simulink model "rlOvertakeTwoCars"  (R2022b)
settings: Solver=ode45  StartTime=0.0  StopTime=inf  FixedStep=0.001  RelTol=5e-3
PreLoadFcn:
  | setUpModel
PostLoadFcn:
  | setUpMain
model workspace (MAT data in the model file):
  firstWarning = 0
  originalScenarioChecksum = 'F73A6DA3C723D3CA73A6F931B7A52A9C'
values from neighbouring files (symbols this model uses):
  accel_vec = (-4:0.5:4)'    [setUpModel.m]
  amax = 3    [setUpMain.m]
  amin = -3    [setUpMain.m]
  dyNorm = [dyNorm 1.1]    [setUpSlipstream.m]
  e1_initial = 0    [setUpMain.m]
  e2_initial = 0    [setUpMain.m]
  L = data.ActorSpecifications.Length    [setUpModel.m]
  psi_o1 = 0.0058 * (pi/180)    (= 0.000101229096616)    [setUpModel.m]
  psi_o2 = 0.3528 *(pi/180)    (= 0.00615752160104)    [setUpModel.m]
  ry = [ry 0]    [setUpSlipstream.m]
  ssSwitch = 1    [setUpSlipstream.m]
  tolpsi = 10 * pi/180    (= 0.174532925199)    [setUpSlipstream.m]
  toly = 1.2*W /2    [setUpSlipstream.m]
  Ts = 0.1    [setUpMPC.m]
  TsRL = Ts    [setUpRLEnv.m]
  umax = 0.3    [setUpMain.m]
  umin = -0.3    [setUpMain.m]
  v_o1 = highSpeed1    (= 35)    [setUpModel.m]
  v_o2 = highSpeed2    (= 36)    [setUpModel.m]
  vel1 = highSpeed1 * ones(length(xlt),length(ylt))    [setUpModel.m]
  vel2 = highSpeed2 * ones(length(xlt),length(ylt))    [setUpModel.m]
  vel_vec = 0:2:20    [setUpModel.m]
  W = data.ActorSpecifications(1,1).Width    [setUpSlipstream.m]
  X_o1 = xRef1(1)    [setUpModel.m]
  X_o2 = xRef2(1)    [setUpModel.m]
  xFollow = [0 x1 xFollow 60]    [setUpSlipstream.m]
  xLead = [0 -x0 xLead]    [setUpSlipstream.m]
  xlt = -250:10:200    [setUpModel.m]
  Y_o1 = yRef1(1)    [setUpModel.m]
  Y_o2 = yRef2(1)    [setUpModel.m]
  yFollow = [c y1 yFollow 1]    [setUpSlipstream.m]
  yLead = [c y0 yLead]    [setUpSlipstream.m]
  ylt = -150:10:100    [setUpModel.m]
undefined symbols (not defined in the file or in its folder): curvature1, curvature2, deg, DiscIntNeverNeededParam, gradbp1, gradbp2, psi, rad, s, v_o, x_colpen, x_o, y_colpen, Z_colpen
libraries: simulink x26, autolibsharedcommon x22, autolibutils x10, autolibshared x10, vehdynlibtirecommon x8, drivingscenarioandsensors x4, autolibpowerinfoutils x4, sharedtransform x4, aerolibconvert2 x2, simulink_extras x2, vehdynlibtire x2, mpcadaslib x1
(part 2 of 8)

== system rlOvertakeTwoCars/Obs // Reward 9-6 ==
  xgap : Inport
  ygap : Inport  Port=2
  v_lead : Inport  Port=3
  v_ego : Inport  Port=4
  v_ref : Inport  Port=5
  e1 : Inport  Port=6
  e2 : Inport  Port=7
  e1dot : Inport  Port=8
  e2dot : Inport  Port=9
  accel : Inport  Port=10
  steer : Inport  Port=11
  collided : Inport  Port=12
  A : Gain  Gain=0
  Abs : Abs  SaturateOnIntegerOverflow=off
  B : Gain  Gain=2000
  Compare To Constant : simulink/Logic and Bit Operations/Compare To Constant  relop=<=  const=6  OutDataTypeStr=boolean
  E : Gain  Gain=2000
  Gain : Gain  Gain=1/TsRL
  Gain1 : Gain  Gain=20
  Gain2 : Gain  Gain=1/TsRL
  Gain3 : Gain  Gain=1/TsRL
  Goto1 : Goto  Commented=on  GotoTag=p_col  TagVisibility=global
  H : Gain
  Integrator : Integrator
  Integrator1 : Integrator
  Integrator2 : Integrator
  Logical Operator1 : Logic  Operator=OR  Inputs=3  AllPortsSameDT=off  OutDataTypeStr=boolean
  Overtaking : Subsystem
  Path following : Subsystem
  Scope : Scope  NumInputPorts=3
  Scope1 : Scope  NumInputPorts=3
  Scope2 : Scope  NumInputPorts=2
  Subsystem : Subsystem
  Subsystem2 : Subsystem
  Sum : Sum  Inputs=--++
  Sum1 : Sum  Inputs=+++
  Sum2 : Sum
  Zone collision penalty : Lookup_n-D  Commented=on  BreakpointsForDimension1=y_colpen  BreakpointsForDimension2=x_colpen  Table=Z_colpen  ExtrapMethod=Clip  InternalRulePriority=Speed  RndMeth=Simplest
      settings: InputPortMap=u0,u1
      mask Display:
      | image("LookupTable.PNG")
      | port_label('input', 1, 'y')
      | port_label('input', 2, 'x')
      | port_label('output', 1, 'p_col')
  obs : Outport  VectorParamsAs1DForOutWhenUnconnected=off
  Reward : Outport  Port=2  VectorParamsAs1DForOutWhenUnconnected=off
  isDone : Outport  Port=3  VectorParamsAs1DForOutWhenUnconnected=off
  tag scope: onTrack=global
  wires:
  Zone collision penalty/1 -> Sum1/3, Goto1/1
  E/1 -> Sum/2
  Subsystem2/2(failCollided) -> Logical Operator1/2, E/1
  Overtaking/1(r_ot) -> Integrator2/1, Scope1/3, Sum1/2
  B/1 -> Sum/4
  Subsystem2/4(overtakeSuccess) -> B/1
  [ry2] -> Overtaking/1(ry)
  Path following/1(r_pf) -> H/1
  e2dot/1 -> Subsystem/6(e2dot)
  e1/1 -> Abs/1, Path following/2(e1), Subsystem/3(e1), Subsystem2/2(e1)
  e2/1 -> Subsystem/4(e2), Path following/3(e2), Subsystem2/3(e2)
  v_lead/1 -> Subsystem/7(v_lead)
  xgap/1 -> Subsystem/8(xgap), Subsystem2/4(xgap), Zone collision penalty/2, Overtaking/2(xgap)
  Subsystem/1(obs) -> obs/1
  e1dot/1 -> Subsystem/5(e1dot)
  Gain1/1 -> Sum/1
  Abs/1 -> Compare To Constant/1
  Compare To Constant/1 -> [onTrack]
  collided/1 -> Subsystem2/5(collided)
  v_ref/1 -> Subsystem/2(v_ref)
  ygap/1 -> Overtaking/3(ygap), Subsystem/9(ygap), Zone collision penalty/1
  Subsystem/2(v_err) -> Path following/1(v_err), Scope2/2
  steer/1 -> Path following/4(steer)
  accel/1 -> Path following/5(accel)
  Logical Operator1/1 -> isDone/1
  v_ego/1 -> Subsystem2/1(v_ego), Scope2/1, Subsystem/1(v_ego)
  Subsystem2/1(fail) -> Logical Operator1/1, Gain1/1
  Subsystem2/3(completeCourse) -> A/1, Logical Operator1/3
  A/1 -> Sum/3
  Sum2/1 -> Reward/1
  Sum/1 -> Sum2/1
  Sum1/1 -> Scope1/1, Integrator/1, Sum2/2
  Gain/1 -> Scope/1
  Integrator/1 -> Gain/1
  Integrator1/1 -> Gain2/1
  Integrator2/1 -> Gain3/1
  Gain2/1 -> Scope/2
  Gain3/1 -> Scope/3
  H/1 -> Integrator1/1, Scope1/2, Sum1/1

== system rlOvertakeTwoCars/Pedal mapping ==
  xdot : Inport
  AccelerationCmd : Inport  Port=2
  2-D Lookup Table : Lookup_n-D  BreakpointsForDimension1=vel_vec  BreakpointsForDimension2=accel_vec  Table=pedal_map'  InternalRulePriority=Speed  RndMeth=Simplest
      settings: InputPortMap=u0,u1
  Dead Zone1 : DeadZone  LowerValue=-0.001  UpperValue=0.001
  Dead Zone2 : DeadZone  LowerValue=-0.001  UpperValue=0.001
  Gain : Gain  Gain=-1
  Saturation : Saturate  UpperLimit=1  LowerLimit=0
  Saturation1 : Saturate  UpperLimit=0  LowerLimit=-1
  Accel : Outport
  Decel : Outport  Port=2
  wires:
  Dead Zone1/1 -> Accel/1  "Accel"
  Dead Zone2/1 -> Decel/1  "Decel"
  xdot/1 -> 2-D Lookup Table/1
  Saturation/1 -> Dead Zone1/1
  AccelerationCmd/1 -> 2-D Lookup Table/2
  2-D Lookup Table/1 -> Saturation/1, Saturation1/1
  Gain/1 -> Dead Zone2/1
  Saturation1/1 -> Gain/1

== system rlOvertakeTwoCars/Powertrain & Driveline ==
  note: needs x4
  note: Vehicle Feedback
  note: Powertrain & Driveline
  note: Brakes
  note: Longitudinal Command Logic
  Acc : Inport
  Decel : Inport  Port=2
  Friction : Inport  Port=3
  VehFdbk : Inport  Port=4
  Brake System : Subsystem
  Brakes and Wheels : Subsystem  TreatAsAtomicUnit=on
      mask Display: image('vdbslibwhls.png');
  Bus Selector1 : BusSelector  OutputSignals=BdyFrm.Forces.Tires.FrntTires.Lft.Fz,BdyFrm.Forces.Tires.FrntTires.Rght.Fz,BdyFrm.Forces.Tires.RearTires.Lft.Fz,BdyFrm.Forces.Tires.RearTires.Rght.Fz
  Bus Selector2 : BusSelector  OutputSignals=BdyFrm.Cg.Vel.xdot  OutputAsBus=on
  Bus Selector3 : BusSelector  OutputSignals=BdyFrm.FrntAxl.Steer.WhlAngFL,BdyFrm.FrntAxl.Steer.WhlAngFR,BdyFrm.RearAxl.Steer.WhlAngRL,BdyFrm.RearAxl.Steer.WhlAngRR  OutputAsBus=on
  Bus Selector4 : BusSelector  OutputSignals=BdyFrm.Cg.AngVel.r
  Bus to Vector : BusToVector
  Constant : Constant  Value=-1
  Constant1 : Constant  Value=-1
  Motor and Differential : Subsystem
  Mux1 : Mux
  Selector : Selector  InputPortWidth=1  IndexOptions=Index vector (dialog)  Indices=[1 1 1 1]  OutputSizes=1
  Signal Specification : SignalSpecification  Unit=km/hr
  Suspension : autolibutils/Cont LPF  wc=10*pi*2  AbsoluteTolerance=auto  aMode=2
  Switch1 : Switch  Criteria=u2 > Threshold  SaturateOnIntegerOverflow=off  InputSameDT=off
  Switch2 : Switch  Criteria=u2 > Threshold  SaturateOnIntegerOverflow=off  InputSameDT=off
  Terminator : Terminator
  Terminator1 : Terminator
  Unit Conversion : UnitConversion
  Vehicle to Tire : Subsystem
  Front Force : Outport  VectorParamsAs1DForOutWhenUnconnected=off
  Rear Force : Outport  Port=2  VectorParamsAs1DForOutWhenUnconnected=off
  wires:
  Vehicle to Tire/2(WhlVel) -> Brakes and Wheels/4(Vy)
  Vehicle to Tire/1(WhlVelx) -> Brakes and Wheels/3(Vx)
  Brakes and Wheels/1(AxlPwr) -> Terminator1/1
  Brakes and Wheels/4(RearF) -> Rear Force/1
  Brakes and Wheels/3(FrontF) -> Front Force/1
  Brakes and Wheels/2(Omega) -> [Omega]
  VehFdbk/1 -> Vehicle to Tire/1(VehFdbk), Bus Selector3/1, Bus Selector1/1, Bus Selector4/1, Bus Selector2/1
  Selector/1 -> Brakes and Wheels/7(YawRate)
  Bus Selector4/1 -> Selector/1  "<r>"
  Friction/1 -> Brakes and Wheels/8(Friction)
  Signal Specification/1 -> Terminator/1
  Unit Conversion/1 -> Signal Specification/1
  Bus Selector2/1 -> Unit Conversion/1
  Brake System/1(Prs) -> Brakes and Wheels/2(BrkPrs)
  Switch2/1 -> Brake System/1(Decc)  "Decc"
  Bus Selector1/4 -> Mux1/4  "<Fz>"
  Bus Selector1/3 -> Mux1/3  "<Fz>"
  Bus Selector1/2 -> Mux1/2  "<Fz>"
  Bus Selector1/1 -> Mux1/1  "<Fz>"
  Suspension/1 -> Brakes and Wheels/6(Fz)
  Mux1/1 -> Suspension/1
  Bus to Vector/1 -> Brakes and Wheels/5(WhlAng), Vehicle to Tire/2(WhlAng)
  Bus Selector3/1 -> Bus to Vector/1
  Acc/1 -> Switch1/3
  Decel/1 -> Switch2/1, Switch2/2, Switch1/2
  Switch1/1 -> Motor and Differential/1(APP)  "Acc"
  Motor and Differential/1(Axle Torque) -> Brakes and Wheels/1(AxlTrq)
  Constant1/1 -> Switch1/1
  [Omega] -> Motor and Differential/2(Omega)  "Omega"
  Constant/1 -> Switch2/3

== system rlOvertakeTwoCars/Powertrain & Driveline Ego ==
  note: needs x4
  note: Vehicle Feedback
  note: Powertrain & Driveline
  note: Brakes
  note: Longitudinal Command Logic
  Acc : Inport
  Decel : Inport  Port=2
  Friction : Inport  Port=3
  VehFdbk : Inport  Port=4
  Brake System : Subsystem
  Brakes and Wheels : Subsystem  TreatAsAtomicUnit=on
      mask Display: image('vdbslibwhls.png');
  Bus Selector1 : BusSelector  OutputSignals=BdyFrm.Forces.Tires.FrntTires.Lft.Fz,BdyFrm.Forces.Tires.FrntTires.Rght.Fz,BdyFrm.Forces.Tires.RearTires.Lft.Fz,BdyFrm.Forces.Tires.RearTires.Rght.Fz
  Bus Selector2 : BusSelector  OutputSignals=BdyFrm.Cg.Vel.xdot  OutputAsBus=on
  Bus Selector3 : BusSelector  OutputSignals=BdyFrm.FrntAxl.Steer.WhlAngFL,BdyFrm.FrntAxl.Steer.WhlAngFR,BdyFrm.RearAxl.Steer.WhlAngRL,BdyFrm.RearAxl.Steer.WhlAngRR  OutputAsBus=on
  Bus Selector4 : BusSelector  OutputSignals=BdyFrm.Cg.AngVel.r
  Bus to Vector : BusToVector
  Constant : Constant  Value=-1
  Constant1 : Constant  Value=-1
  Motor and Differential : Subsystem
  Mux1 : Mux
  Selector : Selector  InputPortWidth=1  IndexOptions=Index vector (dialog)  Indices=[1 1 1 1]  OutputSizes=1
  Signal Specification : SignalSpecification  Unit=km/hr
  Suspension : autolibutils/Cont LPF  wc=10*pi*2  AbsoluteTolerance=auto  aMode=2
  Switch1 : Switch  Criteria=u2 > Threshold  SaturateOnIntegerOverflow=off  InputSameDT=off
  Switch2 : Switch  Criteria=u2 > Threshold  SaturateOnIntegerOverflow=off  InputSameDT=off
  Terminator : Terminator
  Terminator1 : Terminator
  Unit Conversion : UnitConversion
  Vehicle to Tire : Subsystem
  Front Force : Outport  VectorParamsAs1DForOutWhenUnconnected=off
  Rear Force : Outport  Port=2  VectorParamsAs1DForOutWhenUnconnected=off
  wires:
  Vehicle to Tire/2(WhlVel) -> Brakes and Wheels/4(Vy)
  Vehicle to Tire/1(WhlVelx) -> Brakes and Wheels/3(Vx)
  Brakes and Wheels/1(AxlPwr) -> Terminator1/1
  Brakes and Wheels/4(RearF) -> Rear Force/1
  Brakes and Wheels/3(FrontF) -> Front Force/1
  Brakes and Wheels/2(Omega) -> [Omega]
  VehFdbk/1 -> Vehicle to Tire/1(VehFdbk), Bus Selector3/1, Bus Selector1/1, Bus Selector4/1, Bus Selector2/1
  Selector/1 -> Brakes and Wheels/7(YawRate)
  Bus Selector4/1 -> Selector/1  "<r>"
  Friction/1 -> Brakes and Wheels/8(Friction)
  Signal Specification/1 -> Terminator/1
  Unit Conversion/1 -> Signal Specification/1
  Bus Selector2/1 -> Unit Conversion/1
  Brake System/1(Prs) -> Brakes and Wheels/2(BrkPrs)
  Switch2/1 -> Brake System/1(Decc)  "Decc"
  Bus Selector1/4 -> Mux1/4  "<Fz>"
  Bus Selector1/3 -> Mux1/3  "<Fz>"
  Bus Selector1/2 -> Mux1/2  "<Fz>"
  Bus Selector1/1 -> Mux1/1  "<Fz>"
  Suspension/1 -> Brakes and Wheels/6(Fz)
  Mux1/1 -> Suspension/1
  Bus to Vector/1 -> Brakes and Wheels/5(WhlAng), Vehicle to Tire/2(WhlAng)
  Bus Selector3/1 -> Bus to Vector/1
  Acc/1 -> Switch1/3
  Decel/1 -> Switch2/1, Switch2/2, Switch1/2
  Switch1/1 -> Motor and Differential/1(APP)  "Acc"
  Motor and Differential/1(Axle Torque) -> Brakes and Wheels/1(AxlTrq)
  Constant1/1 -> Switch1/1
  [Omega] -> Motor and Differential/2(Omega)  "Omega"
  Constant/1 -> Switch2/3

== system rlOvertakeTwoCars/Relative distance (Ego from Lead) ==
  pos1 : Inport
  psi1 : Inport  Port=2
  pos2 : Inport  Port=3
  Add : Sum  Inputs=-+
  Add1 : Sum  Inputs=-+
  Add2 : Sum
  Add3 : Sum  Inputs=+-
  Demux : Demux  Outputs=2
  Demux1 : Demux  Outputs=2
  Product{,1..3} (4 alike) : Product
  SinCos : Trigonometry  Operator=sincos
  dx : Outport
  dy : Outport  Port=2
  wires:
  Add2/1 -> dx/1
  Product/1 -> Add2/1
  psi1/1 -> SinCos/1
  Demux1/2 -> Add/2  "y2"
  Product3/1 -> Add3/2
  SinCos/1 -> Product1/1, Product3/1
  Add/1 -> Product1/2, Product2/2  "y2-y1"
  Product2/1 -> Add3/1
  SinCos/2 -> Product/1, Product2/1
  Add3/1 -> dy/1
  Demux/1 -> Add1/1  "x1"
  Product1/1 -> Add2/2
  Demux/2 -> Add/1  "y1"
  Demux1/1 -> Add1/2  "x2"
  Add1/1 -> Product3/2, Product/2  "x2-x1"
  pos1/1 -> Demux/1
  pos2/1 -> Demux1/1

== system rlOvertakeTwoCars/Sensor & road ==
  xdot : Inport
  Curvature lookup : Lookup_n-D  NumberOfTableDimensions=1  BreakpointsForDimension1=gradbp2  Table=curvature2  InterpMethod=Cubic spline  ExtrapMethod=Clip  InternalRulePriority=Speed  RndMeth=Simplest
  Error calculation : Subsystem
  Initial lateral deviation : Constant  Value=e1_initial
  Initial relative yaw angle : Constant  Value=e2_initial
  Integrator : Integrator
  Lateral deviation : Outport
  Relative yaw angle : Outport  Port=2
  e1_dot : Outport  Port=3
  e2_dot : Outport  Port=4
  wires:
  Error calculation/1(Lateral deviation) -> Lateral deviation/1
  Curvature lookup/1 -> Error calculation/4(Curvature)  "rho"
  Error calculation/2(Relative yaw angle) -> Relative yaw angle/1
  Initial lateral deviation/1 -> Error calculation/6(Initial lateral deviation)
  xdot/1 -> Error calculation/1(Longitudinal velocity), Integrator/1
  Initial relative yaw angle/1 -> Error calculation/5(Initial relative yaw angle)
  [ydot2] -> Error calculation/2(Lateral velocity)
  Error calculation/3(e1_dot) -> e1_dot/1
  Integrator/1 -> Curvature lookup/1  "distance"
  Error calculation/4(e2_dot) -> e2_dot/1
  [yawrate2] -> Error calculation/3(Yaw rate)

== system rlOvertakeTwoCars/Slipstream enable ==
  psi1 : Inport
  psi2 : Inport  Port=2
  dy : Inport  Port=3
  AND : Logic  Inputs=3  IconShape=distinctive  AllPortsSameDT=off  OutDataTypeStr=boolean
  Abs : Abs  SaturateOnIntegerOverflow=off
  Abs1 : Abs  SaturateOnIntegerOverflow=off
  Add : Sum  Inputs=+-
  Compare To Constant : simulink/Logic and Bit Operations/Compare To Constant  relop=<=  const=tolpsi  OutDataTypeStr=boolean
  Compare To Constant1 : simulink/Logic and Bit Operations/Compare To Constant  relop=<=  const=toly  OutDataTypeStr=boolean
  Constant : Constant  Value=ssSwitch
  Gain : Gain  Gain=1/(W/2)
  tag scope: SsOn=global, dyNorm=global
  wires:
  Abs/1 -> Compare To Constant/1
  dy/1 -> Abs1/1
  Compare To Constant1/1 -> AND/3
  psi2/1 -> Add/1
  Compare To Constant/1 -> AND/2
  psi1/1 -> Add/2
  Gain/1 -> [dyNorm]
  Abs1/1 -> Gain/1, Compare To Constant1/1
  Add/1 -> Abs/1
  Constant/1 -> AND/1
  AND/1 -> [SsOn]

== system rlOvertakeTwoCars/Steering EMA filter ==
  steer : Inport
  Demux3 : Demux  Outputs=2
  Discrete Filter : DiscreteFilter  Numerator=[0.05]  Denominator=[1 0.95]
  Switch : Switch  Criteria=u2 > Threshold  SaturateOnIntegerOverflow=off  InputSameDT=off
  Terminator5 : Terminator
  delta : Outport
  wires:
  steer/1 -> Switch/3, Discrete Filter/1
  [pos2] -> Demux3/1
  Switch/1 -> delta/1
  Discrete Filter/1 -> Switch/1
  Demux3/2 -> Switch/2  "y2"
  Demux3/1 -> Terminator5/1

== system rlOvertakeTwoCars/Stop Logic ==
  distance : Inport
  Constant : Constant
  Constant3 : Constant  Value=0
  Integrator : Integrator
  Switch : Switch  Threshold=gradbp2(end)+20  SaturateOnIntegerOverflow=off  InputSameDT=off
  stop : Outport
  wires:
  Switch/1 -> stop/1
  Constant3/1 -> Switch/3
  distance/1 -> Integrator/1
  Constant/1 -> Switch/1
  Integrator/1 -> Switch/2

== system rlOvertakeTwoCars/Subsystem ==
  In1 : Inport
  Bus Selector : BusSelector  OutputSignals=InertFrm.Cg.Disp.X,InertFrm.Cg.Disp.Y,InertFrm.Cg.Ang.psi,BdyFrm.Cg.Acc.xddot
  Gain1 : Gain  Gain=180/pi
  Mux : Mux  Inputs=3
  Mux1 : Mux  Inputs=2
  Terminator : Terminator
  Transpose : Math  Operator=transpose  SignedPower=on
  pose : Outport
  pos : Outport  Port=2
  wires:
  Mux/1 -> Transpose/1
  In1/1 -> Bus Selector/1
  Bus Selector/1 -> Mux1/1, Mux/1  "<X>"
  Gain1/1 -> Mux/3
  Bus Selector/2 -> Mux1/2, Mux/2  "<Y>"
  Transpose/1 -> pose/1
  Bus Selector/3 -> Gain1/1  "<psi>"
  Bus Selector/4 -> Terminator/1  "<xddot>"
  Mux1/1 -> pos/1

== system rlOvertakeTwoCars/Subsystem1 ==
  In1 : Inport
  Bus Selector : BusSelector  OutputSignals=InertFrm.Cg.Disp.X,InertFrm.Cg.Disp.Y,InertFrm.Cg.Ang.psi,BdyFrm.Cg.Acc.xddot
  Gain1 : Gain  Gain=180/pi
  Mux : Mux  Inputs=3
  Mux1 : Mux  Inputs=2
  Terminator : Terminator
  Transpose : Math  Operator=transpose  SignedPower=on
  pose : Outport
  pos : Outport  Port=2
  wires:
  Mux/1 -> Transpose/1
  In1/1 -> Bus Selector/1
  Bus Selector/1 -> Mux1/1, Mux/1  "<X>"
  Gain1/1 -> Mux/3
  Bus Selector/2 -> Mux1/2, Mux/2  "<Y>"
  Transpose/1 -> pose/1
  Bus Selector/3 -> Gain1/1  "<psi>"
  Bus Selector/4 -> Terminator/1  "<xddot>"
  Mux1/1 -> pos/1

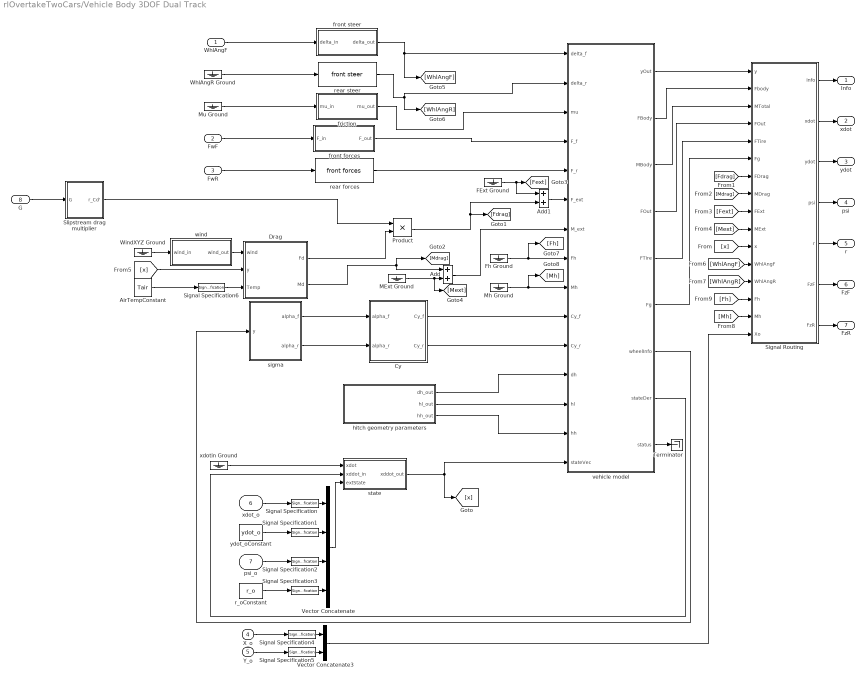
== system rlOvertakeTwoCars/Vehicle Body 3DOF Dual Track ==
  WhlAngF : Inport
  FwF : Inport  Port=2
  FwR : Inport  Port=3
  X_o : Inport  Port=4
  Y_o : Inport  Port=5
  xdot_o : Inport  Port=6
  psi_o : Inport  Port=7
  G : Inport  Port=8
  Add : Sum
  Add1 : Sum
  AirTempConstant : Constant  Value=Tair
  Cy : Subsystem  Variant=on  VariantControlMode=label  LabelModeActiveChoice=2
  Drag : Subsystem
  FExt Ground : Ground
  Fh Ground : Ground
  MExt Ground : Ground
  Mh Ground : Ground
  Mu Ground : Ground
  Product : Product
  Signal Routing : Subsystem  Variant=on  VariantControlMode=label  LabelModeActiveChoice=1
  Signal Specification : SignalSpecification  Unit=m/s
  Signal Specification1 : SignalSpecification  Unit=m/s
  Signal Specification2 : SignalSpecification  Unit=rad
  Signal Specification3 : SignalSpecification  Unit=rad/s
  Signal Specification4 : SignalSpecification  Unit=m
  Signal Specification5 : SignalSpecification  Unit=m
  Signal Specification6 : SignalSpecification  Unit=K
  Slipstream drag multiplier : Subsystem
  Terminator : Terminator
  Vector Concatenate : Concatenate  NumInputs=4
  Vector Concatenate3 : Concatenate
  WhlAngR Ground : Ground
  WindXYZ Ground : Ground
  friction : Subsystem  Variant=on  VariantControlMode=label  LabelModeActiveChoice=2
  front forces : Subsystem  Variant=on  VariantControlMode=label  LabelModeActiveChoice=5
  front steer : Subsystem  Variant=on  VariantControlMode=label  LabelModeActiveChoice=3
  hitch geometry parameters : Subsystem  Variant=on  VariantControlMode=label  LabelModeActiveChoice=3
  r_oConstant : Constant  Value=r_o
  rear forces : autolibshared/Vehicle Body 3DOF Single Track/front forces  SystemSampleTime=-1  LabelModeActiveChoice=5  VariantActivationTime=update diagram  Latency=0  AutoFrameSizeCalculation=off
  rear steer : autolibshared/Vehicle Body 3DOF Single Track/front steer  SystemSampleTime=-1  LabelModeActiveChoice=2  VariantActivationTime=update diagram  Latency=0  AutoFrameSizeCalculation=off
  sigma : Subsystem  Variant=on  VariantControlMode=label  LabelModeActiveChoice=2
  state : Subsystem  Variant=on  VariantControlMode=label  LabelModeActiveChoice=0
  vehicle model : MATLAB Function  TreatAsAtomicUnit=on
  wind : Subsystem  Variant=on  VariantControlMode=label  LabelModeActiveChoice=0
  xdotin Ground : Ground
  ydot_oConstant : Constant  Value=ydot_o
  Info : Outport  VectorParamsAs1DForOutWhenUnconnected=off
  xdot : Outport  Port=2  VectorParamsAs1DForOutWhenUnconnected=off
  ydot : Outport  Port=3  VectorParamsAs1DForOutWhenUnconnected=off
  psi : Outport  Port=4  VectorParamsAs1DForOutWhenUnconnected=off
  r : Outport  Port=5  VectorParamsAs1DForOutWhenUnconnected=off
  FzF : Outport  Port=6  VectorParamsAs1DForOutWhenUnconnected=off
  FzR : Outport  Port=7  VectorParamsAs1DForOutWhenUnconnected=off
  wires:
  AirTempConstant/1 -> Signal Specification6/1
  [Fh] -> Signal Routing/14(Fh)
  [Mh] -> Signal Routing/15(Mh)
  hitch geometry parameters/3(hh_out) -> vehicle model/14(hh)
  hitch geometry parameters/2(hl_out) -> vehicle model/13(hl)
  hitch geometry parameters/1(dh_out) -> vehicle model/12(dh)
  Mh Ground/1 -> [Mh], vehicle model/9(Mh)
  Fh Ground/1 -> [Fh], vehicle model/8(Fh)
  MExt Ground/1 -> Add/2, [Mext]
  FwR/1 -> rear forces/1
  FwF/1 -> front forces/1(F_in)
  xdotin Ground/1 -> state/1(xdot)
  Signal Specification6/1 -> Drag/3(Temp)
  Signal Specification5/1 -> Vector Concatenate3/2
  Signal Specification4/1 -> Vector Concatenate3/1
  Vector Concatenate3/1 -> Signal Routing/16(Xo)
  Signal Specification2/1 -> Vector Concatenate/3
  Signal Specification3/1 -> Vector Concatenate/4
  r_oConstant/1 -> Signal Specification3/1
  Signal Specification1/1 -> Vector Concatenate/2
  ydot_oConstant/1 -> Signal Specification1/1
  Signal Specification/1 -> Vector Concatenate/1
  Vector Concatenate/1 -> state/3(extState)
  [WhlAngR] -> Signal Routing/13(WhlAngR)
  [WhlAngF] -> Signal Routing/12(WhlAngF)
  Signal Routing/4(psi) -> psi/1
  Mu Ground/1 -> friction/1(mu_in)
  WhlAngR Ground/1 -> rear steer/1
  WhlAngF/1 -> front steer/1(delta_in)
  [x] -> Drag/2(y)
  Product/1 -> Add1/2, [Fdrag]
  wind/1(wind_out) -> Drag/1(wind)
  Drag/2(Md) -> [Mdrag], Add/1
  rear forces/1 -> vehicle model/5(F_r)
  front forces/1(F_out) -> vehicle model/4(F_f)
  vehicle model/7(wheelInfo) -> sigma/1(y)
  Signal Routing/1(Info) -> Info/1
  sigma/2(alpha_r) -> Cy/2(alpha_r)
  sigma/1(alpha_f) -> Cy/1(alpha_f)
  rear steer/1 -> vehicle model/2(delta_r), [WhlAngR]
  front steer/1(delta_out) -> [WhlAngF], vehicle model/1(delta_f)
  Cy/2(Cy_r) -> vehicle model/11(Cy_r)
  Cy/1(Cy_f) -> vehicle model/10(Cy_f)
  friction/1(mu_out) -> vehicle model/3(mu)
  vehicle model/8(stateDer) -> state/2(xddot_in)
  vehicle model/1(yOut) -> Signal Routing/1(y)
  Signal Routing/3(ydot) -> ydot/1
  Signal Routing/5(r) -> r/1
  Signal Routing/6(FzF) -> FzF/1
  Signal Routing/7(FzR) -> FzR/1
  Signal Routing/2(xdot) -> xdot/1
  vehicle model/4(FOut) -> Signal Routing/4(FOut)
  state/1(xddot_out) -> vehicle model/15(stateVec), [x]
  [x] -> Signal Routing/11(x)
  vehicle model/9(status) -> Terminator/1
  vehicle model/5(FTire) -> Signal Routing/5(FTire)
  vehicle model/6(Fg) -> Signal Routing/6(Fg)
  [Fext] -> Signal Routing/9(FExt)
  [Fdrag] -> Signal Routing/7(FDrag)
  [Mdrag] -> Signal Routing/8(MDrag)
  [Mext] -> Signal Routing/10(MExt)
  vehicle model/2(FBody) -> Signal Routing/2(Fbody)
  vehicle model/3(MBody) -> Signal Routing/3(MTotal)
  Add/1 -> vehicle model/7(M_ext)
  Add1/1 -> vehicle model/6(F_ext)
  X_o/1 -> Signal Specification4/1
  Y_o/1 -> Signal Specification5/1
  psi_o/1 -> Signal Specification2/1
  xdot_o/1 -> Signal Specification/1
  FExt Ground/1 -> [Fext], Add1/1
  WindXYZ Ground/1 -> wind/1(wind_in)
  Drag/1(Fd) -> Product/2
  G/1 -> Slipstream drag multiplier/1(G)
  Slipstream drag multiplier/1(r_Cd') -> Product/1

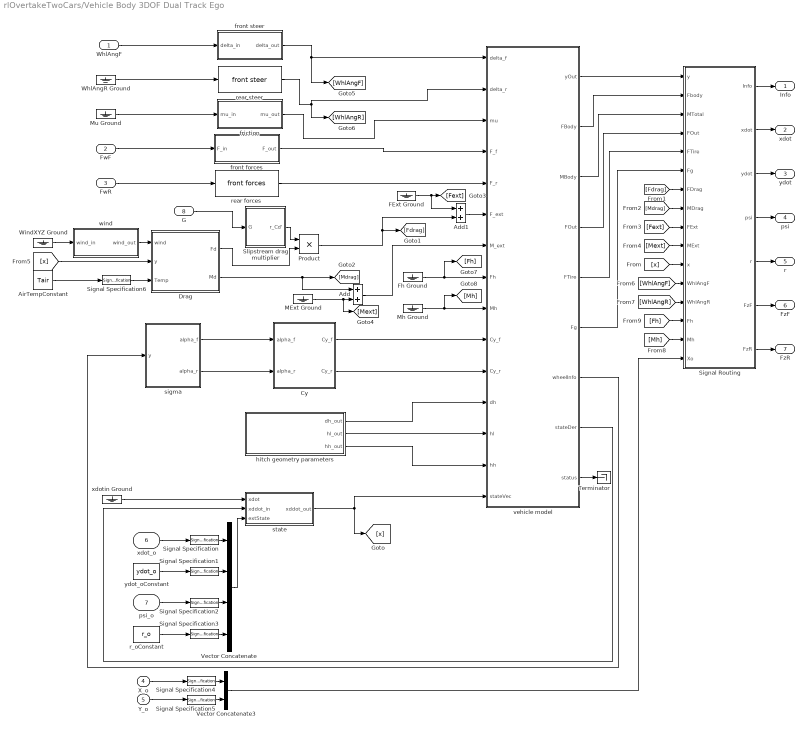
== system rlOvertakeTwoCars/Vehicle Body 3DOF Dual Track Ego ==
  WhlAngF : Inport
  FwF : Inport  Port=2
  FwR : Inport  Port=3
  X_o : Inport  Port=4
  Y_o : Inport  Port=5
  xdot_o : Inport  Port=6
  psi_o : Inport  Port=7
  G : Inport  Port=8
  Add : Sum
  Add1 : Sum
  AirTempConstant : Constant  Value=Tair
  Cy : Subsystem  Variant=on  VariantControlMode=label  LabelModeActiveChoice=2
  Drag : Subsystem
  FExt Ground : Ground
  Fh Ground : Ground
  MExt Ground : Ground
  Mh Ground : Ground
  Mu Ground : Ground
  Product : Product
  Signal Routing : Subsystem  Variant=on  VariantControlMode=label  LabelModeActiveChoice=1
  Signal Specification : SignalSpecification  Unit=m/s
  Signal Specification1 : SignalSpecification  Unit=m/s
  Signal Specification2 : SignalSpecification  Unit=rad
  Signal Specification3 : SignalSpecification  Unit=rad/s
  Signal Specification4 : SignalSpecification  Unit=m
  Signal Specification5 : SignalSpecification  Unit=m
  Signal Specification6 : SignalSpecification  Unit=K
  Slipstream drag multiplier : Subsystem
  Terminator : Terminator
  Vector Concatenate : Concatenate  NumInputs=4
  Vector Concatenate3 : Concatenate
  WhlAngR Ground : Ground
  WindXYZ Ground : Ground
  friction : Subsystem  Variant=on  VariantControlMode=label  LabelModeActiveChoice=2
  front forces : Subsystem  Variant=on  VariantControlMode=label  LabelModeActiveChoice=5
  front steer : Subsystem  Variant=on  VariantControlMode=label  LabelModeActiveChoice=3
  hitch geometry parameters : Subsystem  Variant=on  VariantControlMode=label  LabelModeActiveChoice=3
  r_oConstant : Constant  Value=r_o
  rear forces : autolibshared/Vehicle Body 3DOF Single Track/front forces  SystemSampleTime=-1  LabelModeActiveChoice=5  VariantActivationTime=update diagram  Latency=0  AutoFrameSizeCalculation=off
  rear steer : autolibshared/Vehicle Body 3DOF Single Track/front steer  SystemSampleTime=-1  LabelModeActiveChoice=2  VariantActivationTime=update diagram  Latency=0  AutoFrameSizeCalculation=off
  sigma : Subsystem  Variant=on  VariantControlMode=label  LabelModeActiveChoice=2
  state : Subsystem  Variant=on  VariantControlMode=label  LabelModeActiveChoice=0
  vehicle model : MATLAB Function  TreatAsAtomicUnit=on
  wind : Subsystem  Variant=on  VariantControlMode=label  LabelModeActiveChoice=0
  xdotin Ground : Ground
  ydot_oConstant : Constant  Value=ydot_o
  Info : Outport  VectorParamsAs1DForOutWhenUnconnected=off
  xdot : Outport  Port=2  VectorParamsAs1DForOutWhenUnconnected=off
  ydot : Outport  Port=3  VectorParamsAs1DForOutWhenUnconnected=off
  psi : Outport  Port=4  VectorParamsAs1DForOutWhenUnconnected=off
  r : Outport  Port=5  VectorParamsAs1DForOutWhenUnconnected=off
  FzF : Outport  Port=6  VectorParamsAs1DForOutWhenUnconnected=off
  FzR : Outport  Port=7  VectorParamsAs1DForOutWhenUnconnected=off
  wires:
  AirTempConstant/1 -> Signal Specification6/1
  [Fh] -> Signal Routing/14(Fh)
  [Mh] -> Signal Routing/15(Mh)
  hitch geometry parameters/3(hh_out) -> vehicle model/14(hh)
  hitch geometry parameters/2(hl_out) -> vehicle model/13(hl)
  hitch geometry parameters/1(dh_out) -> vehicle model/12(dh)
  Mh Ground/1 -> [Mh], vehicle model/9(Mh)
  Fh Ground/1 -> [Fh], vehicle model/8(Fh)
  MExt Ground/1 -> Add/2, [Mext]
  FwR/1 -> rear forces/1
  FwF/1 -> front forces/1(F_in)
  xdotin Ground/1 -> state/1(xdot)
  Signal Specification6/1 -> Drag/3(Temp)
  Signal Specification5/1 -> Vector Concatenate3/2
  Signal Specification4/1 -> Vector Concatenate3/1
  Vector Concatenate3/1 -> Signal Routing/16(Xo)
  Signal Specification2/1 -> Vector Concatenate/3
  Signal Specification3/1 -> Vector Concatenate/4
  r_oConstant/1 -> Signal Specification3/1
  Signal Specification1/1 -> Vector Concatenate/2
  ydot_oConstant/1 -> Signal Specification1/1
  Signal Specification/1 -> Vector Concatenate/1
  Vector Concatenate/1 -> state/3(extState)
  [WhlAngR] -> Signal Routing/13(WhlAngR)
  [WhlAngF] -> Signal Routing/12(WhlAngF)
  Signal Routing/4(psi) -> psi/1
  Mu Ground/1 -> friction/1(mu_in)
  WhlAngR Ground/1 -> rear steer/1
  WhlAngF/1 -> front steer/1(delta_in)
  [x] -> Drag/2(y)
  Product/1 -> Add1/2, [Fdrag]
  wind/1(wind_out) -> Drag/1(wind)
  Drag/2(Md) -> Add/1, [Mdrag]
  rear forces/1 -> vehicle model/5(F_r)
  front forces/1(F_out) -> vehicle model/4(F_f)
  vehicle model/7(wheelInfo) -> sigma/1(y)
  Signal Routing/1(Info) -> Info/1
  sigma/2(alpha_r) -> Cy/2(alpha_r)
  sigma/1(alpha_f) -> Cy/1(alpha_f)
  rear steer/1 -> vehicle model/2(delta_r), [WhlAngR]
  front steer/1(delta_out) -> [WhlAngF], vehicle model/1(delta_f)
  Cy/2(Cy_r) -> vehicle model/11(Cy_r)
  Cy/1(Cy_f) -> vehicle model/10(Cy_f)
  friction/1(mu_out) -> vehicle model/3(mu)
  vehicle model/8(stateDer) -> state/2(xddot_in)
  vehicle model/1(yOut) -> Signal Routing/1(y)
  Signal Routing/3(ydot) -> ydot/1
  Signal Routing/5(r) -> r/1
  Signal Routing/6(FzF) -> FzF/1
  Signal Routing/7(FzR) -> FzR/1
  Signal Routing/2(xdot) -> xdot/1
  vehicle model/4(FOut) -> Signal Routing/4(FOut)
  state/1(xddot_out) -> vehicle model/15(stateVec), [x]
  [x] -> Signal Routing/11(x)
  vehicle model/9(status) -> Terminator/1
  vehicle model/5(FTire) -> Signal Routing/5(FTire)
  vehicle model/6(Fg) -> Signal Routing/6(Fg)
  [Fext] -> Signal Routing/9(FExt)
  [Fdrag] -> Signal Routing/7(FDrag)
  [Mdrag] -> Signal Routing/8(MDrag)
  [Mext] -> Signal Routing/10(MExt)
  vehicle model/2(FBody) -> Signal Routing/2(Fbody)
  vehicle model/3(MBody) -> Signal Routing/3(MTotal)
  Add/1 -> vehicle model/7(M_ext)
  Add1/1 -> vehicle model/6(F_ext)
  X_o/1 -> Signal Specification4/1
  Y_o/1 -> Signal Specification5/1
  psi_o/1 -> Signal Specification2/1
  xdot_o/1 -> Signal Specification/1
  FExt Ground/1 -> [Fext], Add1/1
  WindXYZ Ground/1 -> wind/1(wind_in)
  Drag/1(Fd) -> Product/2
  G/1 -> Slipstream drag multiplier/1(G)
  Slipstream drag multiplier/1(r_Cd') -> Product/1

== system rlOvertakeTwoCars/Collision Detector/Corner and car centre 1 ==
  psi1 : Inport
  pos1 : Inport  Port=2
  Add : Sum
  Add1 : Sum
  Add10 : Sum  Inputs=++-
  Add11 : Sum  Inputs=+++
  Add12 : Sum  Inputs=+++
  Add13 : Sum  Inputs=++-
  Add6 : Sum  Inputs=+--
  Add7 : Sum  Inputs=+-+
  Add8 : Sum  Inputs=+-+
  Add9 : Sum  Inputs=+--
  Demux : Demux  Outputs=2
  Gain : Gain  Gain=L/2-1
  Gain2 : Gain  Gain=L/2-1
  Gain3 : Gain  Gain=L/2
  Gain4 : Gain  Gain=L/2
  Gain5 : Gain  Gain=W/2
  Gain6 : Gain  Gain=W/2
  Mux{1..5} (5 alike) : Mux  Inputs=2
  Mux6 : Mux
  SinCos : Trigonometry  Operator=sincos
  c1 : Outport
  corners_v1 : Outport  Port=2
  wires:
  Demux/1 -> Add1/2  "x1"
  Add12/1 -> Mux5/1
  Add13/1 -> Mux5/2
  Add6/1 -> Mux2/1
  Mux2/1 -> Mux6/1
  psi1/1 -> SinCos/1
  Add/1 -> Mux1/2, Add13/1, Add11/1, Add9/1, Add7/1  "yc"
  Mux3/1 -> Mux6/2
  Mux6/1 -> corners_v1/1
  Mux4/1 -> Mux6/3
  Gain3/1 -> Add12/2, Add8/2, Add6/2, Add10/2
  Add11/1 -> Mux4/2
  Add7/1 -> Mux2/2
  Gain6/1 -> Add8/3, Add6/3, Add10/3, Add12/3
  Add9/1 -> Mux3/2
  Add1/1 -> Add12/1, Add10/1, Add8/1, Mux1/1, Add6/1  "xc"
  SinCos/1 -> Gain6/1, Gain4/1, Gain/1  "s"
  Add8/1 -> Mux3/1
  Demux/2 -> Add/2  "y1"
  Gain/1 -> Add1/1
  SinCos/2 -> Gain5/1, Gain3/1, Gain2/1  "c"
  Mux5/1 -> Mux6/4
  Gain2/1 -> Add/1
  Add10/1 -> Mux4/1
  Gain4/1 -> Add13/2, Add11/2, Add9/2, Add7/2
  Gain5/1 -> Add11/3, Add9/3, Add7/3, Add13/3
  Mux1/1 -> c1/1
  pos1/1 -> Demux/1

== system rlOvertakeTwoCars/Collision Detector/Corner and car centre 2 ==
  psi2 : Inport
  pos2 : Inport  Port=2
  Add : Sum
  Add1 : Sum
  Add10 : Sum  Inputs=++-
  Add11 : Sum  Inputs=+++
  Add12 : Sum  Inputs=+++
  Add13 : Sum  Inputs=++-
  Add6 : Sum  Inputs=+--
  Add7 : Sum  Inputs=+-+
  Add8 : Sum  Inputs=+-+
  Add9 : Sum  Inputs=+--
  Demux : Demux  Outputs=2
  Gain : Gain  Gain=L/2-1
  Gain2 : Gain  Gain=L/2-1
  Gain3 : Gain  Gain=L/2
  Gain4 : Gain  Gain=L/2
  Gain5 : Gain  Gain=W/2
  Gain6 : Gain  Gain=W/2
  Mux{1..5} (5 alike) : Mux  Inputs=2
  Mux6 : Mux
  SinCos : Trigonometry  Operator=sincos
  c2 : Outport
  corners_v2 : Outport  Port=2
  wires:
  Demux/1 -> Add1/2
  Add12/1 -> Mux5/1
  Add13/1 -> Mux5/2
  Add6/1 -> Mux2/1
  Mux2/1 -> Mux6/1
  psi2/1 -> SinCos/1
  Add/1 -> Mux1/2, Add13/1, Add11/1, Add9/1, Add7/1  "yc"
  Mux3/1 -> Mux6/2
  Mux6/1 -> corners_v2/1
  Mux4/1 -> Mux6/3
  Gain3/1 -> Add12/2, Add8/2, Add6/2, Add10/2
  Add11/1 -> Mux4/2
  Add7/1 -> Mux2/2
  Gain6/1 -> Add8/3, Add6/3, Add10/3, Add12/3
  Add9/1 -> Mux3/2
  Add1/1 -> Add12/1, Add10/1, Add8/1, Mux1/1, Add6/1  "xc"
  SinCos/1 -> Gain6/1, Gain4/1, Gain/1  "s"
  Add8/1 -> Mux3/1
  Demux/2 -> Add/2
  Gain/1 -> Add1/1
  SinCos/2 -> Gain5/1, Gain3/1, Gain2/1  "c"
  Mux5/1 -> Mux6/4
  Gain2/1 -> Add/1
  Add10/1 -> Mux4/1
  Gain4/1 -> Add13/2, Add11/2, Add9/2, Add7/2
  Gain5/1 -> Add11/3, Add9/3, Add7/3, Add13/3
  Mux1/1 -> c2/1
  pos2/1 -> Demux/1

== system rlOvertakeTwoCars/Collision Detector/Subsystem10 ==
  psi1 : Inport
  c1 : Inport  Port=2
  v2cor3 : Inport  Port=3
  Abs : Abs  SaturateOnIntegerOverflow=off
  Abs1 : Abs  SaturateOnIntegerOverflow=off
  Add : Sum  Inputs=-+
  Add1 : Sum  Inputs=-+
  Add2 : Sum  Inputs=+-
  Add3 : Sum
  Compare To Constant : simulink/Logic and Bit Operations/Compare To Constant  relop=>  const=L/2  OutDataTypeStr=boolean
  Compare To Constant1 : simulink/Logic and Bit Operations/Compare To Constant  relop=>  const=W/2  OutDataTypeStr=boolean
  Demux1 : Demux  Outputs=2
  Demux2 : Demux  Outputs=2
  Gain : Gain  Gain=-1
  NOT : Logic  Operator=NOT  IconShape=distinctive  AllPortsSameDT=off  OutDataTypeStr=boolean
  OR : Logic  Operator=OR  IconShape=distinctive  AllPortsSameDT=off  OutDataTypeStr=boolean
  Product{,1..3} (4 alike) : Product
  SinCos : Trigonometry  Operator=sincos
  collided : Outport
  wires:
  Demux2/1 -> Add1/1
  OR/1 -> NOT/1
  c1/1 -> Demux2/1
  Add1/1 -> Product2/1, Product/1  "dx"
  SinCos/1 -> Product2/2, Product1/2  "s"
  Demux1/1 -> Add1/2  "point0"
  Abs1/1 -> Compare To Constant1/1
  Compare To Constant1/1 -> OR/2
  Demux1/2 -> Add/2  "point1"
  NOT/1 -> collided/1
  Abs/1 -> Compare To Constant/1
  Demux2/2 -> Add/1
  Product/1 -> Add2/1
  v2cor3/1 -> Demux1/1
  psi1/1 -> Gain/1
  Gain/1 -> SinCos/1
  Product2/1 -> Add3/1
  Product3/1 -> Add3/2
  Compare To Constant/1 -> OR/1
  SinCos/2 -> Product3/2, Product/2  "c"
  Add2/1 -> Abs/1  "rot_dx"
  Add3/1 -> Abs1/1  "rot_dy"
  Product1/1 -> Add2/2
  Add/1 -> Product1/1, Product3/1  "dy"

== system rlOvertakeTwoCars/Collision Detector/Subsystem11 ==
  psi1 : Inport
  c1 : Inport  Port=2
  v2cor4 : Inport  Port=3
  Abs : Abs  SaturateOnIntegerOverflow=off
  Abs1 : Abs  SaturateOnIntegerOverflow=off
  Add : Sum  Inputs=-+
  Add1 : Sum  Inputs=-+
  Add2 : Sum  Inputs=+-
  Add3 : Sum
  Compare To Constant : simulink/Logic and Bit Operations/Compare To Constant  relop=>  const=L/2  OutDataTypeStr=boolean
  Compare To Constant1 : simulink/Logic and Bit Operations/Compare To Constant  relop=>  const=W/2  OutDataTypeStr=boolean
  Demux1 : Demux  Outputs=2
  Demux2 : Demux  Outputs=2
  Gain : Gain  Gain=-1
  NOT : Logic  Operator=NOT  IconShape=distinctive  AllPortsSameDT=off  OutDataTypeStr=boolean
  OR : Logic  Operator=OR  IconShape=distinctive  AllPortsSameDT=off  OutDataTypeStr=boolean
  Product{,1..3} (4 alike) : Product
  SinCos : Trigonometry  Operator=sincos
  collided : Outport
  wires:
  Demux2/1 -> Add1/1
  OR/1 -> NOT/1
  c1/1 -> Demux2/1
  Add1/1 -> Product2/1, Product/1  "dx"
  SinCos/1 -> Product2/2, Product1/2  "s"
  Demux1/1 -> Add1/2  "point0"
  Abs1/1 -> Compare To Constant1/1
  Compare To Constant1/1 -> OR/2
  Demux1/2 -> Add/2  "point1"
  NOT/1 -> collided/1
  Abs/1 -> Compare To Constant/1
  Demux2/2 -> Add/1
  Product/1 -> Add2/1
  v2cor4/1 -> Demux1/1
  psi1/1 -> Gain/1
  Gain/1 -> SinCos/1
  Product2/1 -> Add3/1
  Product3/1 -> Add3/2
  Compare To Constant/1 -> OR/1
  SinCos/2 -> Product3/2, Product/2  "c"
  Add2/1 -> Abs/1  "rot_dx"
  Add3/1 -> Abs1/1  "rot_dy"
  Product1/1 -> Add2/2
  Add/1 -> Product1/1, Product3/1  "dy"

== system rlOvertakeTwoCars/Collision Detector/Subsystem3 ==
  psi2 : Inport
  c2 : Inport  Port=2
  v1cor1 : Inport  Port=3
  Abs : Abs  SaturateOnIntegerOverflow=off
  Abs1 : Abs  SaturateOnIntegerOverflow=off
  Add : Sum  Inputs=-+
  Add1 : Sum  Inputs=-+
  Add2 : Sum  Inputs=+-
  Add3 : Sum
  Compare To Constant : simulink/Logic and Bit Operations/Compare To Constant  relop=>  const=L/2  OutDataTypeStr=boolean
  Compare To Constant1 : simulink/Logic and Bit Operations/Compare To Constant  relop=>  const=W/2  OutDataTypeStr=boolean
  Demux1 : Demux  Outputs=2
  Demux2 : Demux  Outputs=2
  Gain : Gain  Gain=-1
  NOT : Logic  Operator=NOT  IconShape=distinctive  AllPortsSameDT=off  OutDataTypeStr=boolean
  OR : Logic  Operator=OR  IconShape=distinctive  AllPortsSameDT=off  OutDataTypeStr=boolean
  Product{,1..3} (4 alike) : Product
  SinCos : Trigonometry  Operator=sincos
  collided : Outport
  wires:
  Demux2/1 -> Add1/1
  OR/1 -> NOT/1
  c2/1 -> Demux2/1
  Add1/1 -> Product2/1, Product/1  "dx"
  SinCos/1 -> Product2/2, Product1/2  "s"
  Demux1/1 -> Add1/2  "point0"
  Abs1/1 -> Compare To Constant1/1
  Compare To Constant1/1 -> OR/2
  Demux1/2 -> Add/2  "point1"
  NOT/1 -> collided/1
  Abs/1 -> Compare To Constant/1
  Demux2/2 -> Add/1
  Product/1 -> Add2/1
  v1cor1/1 -> Demux1/1
  psi2/1 -> Gain/1
  Gain/1 -> SinCos/1
  Product2/1 -> Add3/1
  Product3/1 -> Add3/2
  Compare To Constant/1 -> OR/1
  SinCos/2 -> Product3/2, Product/2  "c"
  Add2/1 -> Abs/1  "rot_dx"
  Add3/1 -> Abs1/1  "rot_dy"
  Product1/1 -> Add2/2
  Add/1 -> Product1/1, Product3/1  "dy"

== system rlOvertakeTwoCars/Collision Detector/Subsystem5 ==
  psi2 : Inport
  c2 : Inport  Port=2
  v1cor2 : Inport  Port=3
  Abs : Abs  SaturateOnIntegerOverflow=off
  Abs1 : Abs  SaturateOnIntegerOverflow=off
  Add : Sum  Inputs=-+
  Add1 : Sum  Inputs=-+
  Add2 : Sum  Inputs=+-
  Add3 : Sum
  Compare To Constant : simulink/Logic and Bit Operations/Compare To Constant  relop=>  const=L/2  OutDataTypeStr=boolean
  Compare To Constant1 : simulink/Logic and Bit Operations/Compare To Constant  relop=>  const=W/2  OutDataTypeStr=boolean
  Demux1 : Demux  Outputs=2
  Demux2 : Demux  Outputs=2
  Gain : Gain  Gain=-1
  NOT : Logic  Operator=NOT  IconShape=distinctive  AllPortsSameDT=off  OutDataTypeStr=boolean
  OR : Logic  Operator=OR  IconShape=distinctive  AllPortsSameDT=off  OutDataTypeStr=boolean
  Product{,1..3} (4 alike) : Product
  SinCos : Trigonometry  Operator=sincos
  collided : Outport
  wires:
  Demux2/1 -> Add1/1
  OR/1 -> NOT/1
  c2/1 -> Demux2/1
  Add1/1 -> Product2/1, Product/1  "dx"
  SinCos/1 -> Product2/2, Product1/2  "s"
  Demux1/1 -> Add1/2  "point0"
  Abs1/1 -> Compare To Constant1/1
  Compare To Constant1/1 -> OR/2
  Demux1/2 -> Add/2  "point1"
  NOT/1 -> collided/1
  Abs/1 -> Compare To Constant/1
  Demux2/2 -> Add/1
  Product/1 -> Add2/1
  v1cor2/1 -> Demux1/1
  psi2/1 -> Gain/1
  Gain/1 -> SinCos/1
  Product2/1 -> Add3/1
  Product3/1 -> Add3/2
  Compare To Constant/1 -> OR/1
  SinCos/2 -> Product3/2, Product/2  "c"
  Add2/1 -> Abs/1  "rot_dx"
  Add3/1 -> Abs1/1  "rot_dy"
  Product1/1 -> Add2/2
  Add/1 -> Product1/1, Product3/1  "dy"

== system rlOvertakeTwoCars/Collision Detector/Subsystem6 ==
  psi2 : Inport
  c2 : Inport  Port=2
  v1cor3 : Inport  Port=3
  Abs : Abs  SaturateOnIntegerOverflow=off
  Abs1 : Abs  SaturateOnIntegerOverflow=off
  Add : Sum  Inputs=-+
  Add1 : Sum  Inputs=-+
  Add2 : Sum  Inputs=+-
  Add3 : Sum
  Compare To Constant : simulink/Logic and Bit Operations/Compare To Constant  relop=>  const=L/2  OutDataTypeStr=boolean
  Compare To Constant1 : simulink/Logic and Bit Operations/Compare To Constant  relop=>  const=W/2  OutDataTypeStr=boolean
  Demux1 : Demux  Outputs=2
  Demux2 : Demux  Outputs=2
  Gain : Gain  Gain=-1
  NOT : Logic  Operator=NOT  IconShape=distinctive  AllPortsSameDT=off  OutDataTypeStr=boolean
  OR : Logic  Operator=OR  IconShape=distinctive  AllPortsSameDT=off  OutDataTypeStr=boolean
  Product{,1..3} (4 alike) : Product
  SinCos : Trigonometry  Operator=sincos
  collided : Outport
  wires:
  Demux2/1 -> Add1/1
  OR/1 -> NOT/1
  c2/1 -> Demux2/1
  Add1/1 -> Product2/1, Product/1  "dx"
  SinCos/1 -> Product2/2, Product1/2  "s"
  Demux1/1 -> Add1/2  "point0"
  Abs1/1 -> Compare To Constant1/1
  Compare To Constant1/1 -> OR/2
  Demux1/2 -> Add/2  "point1"
  NOT/1 -> collided/1
  Abs/1 -> Compare To Constant/1
  Demux2/2 -> Add/1
  Product/1 -> Add2/1
  v1cor3/1 -> Demux1/1
  psi2/1 -> Gain/1
  Gain/1 -> SinCos/1
  Product2/1 -> Add3/1
  Product3/1 -> Add3/2
  Compare To Constant/1 -> OR/1
  SinCos/2 -> Product3/2, Product/2  "c"
  Add2/1 -> Abs/1  "rot_dx"
  Add3/1 -> Abs1/1  "rot_dy"
  Product1/1 -> Add2/2
  Add/1 -> Product1/1, Product3/1  "dy"

== system rlOvertakeTwoCars/Collision Detector/Subsystem7 ==
  psi2 : Inport
  c2 : Inport  Port=2
  v1cor4 : Inport  Port=3
  Abs : Abs  SaturateOnIntegerOverflow=off
  Abs1 : Abs  SaturateOnIntegerOverflow=off
  Add : Sum  Inputs=-+
  Add1 : Sum  Inputs=-+
  Add2 : Sum  Inputs=+-
  Add3 : Sum
  Compare To Constant : simulink/Logic and Bit Operations/Compare To Constant  relop=>  const=L/2  OutDataTypeStr=boolean
  Compare To Constant1 : simulink/Logic and Bit Operations/Compare To Constant  relop=>  const=W/2  OutDataTypeStr=boolean
  Demux1 : Demux  Outputs=2
  Demux2 : Demux  Outputs=2
  Gain : Gain  Gain=-1
  NOT : Logic  Operator=NOT  IconShape=distinctive  AllPortsSameDT=off  OutDataTypeStr=boolean
  OR : Logic  Operator=OR  IconShape=distinctive  AllPortsSameDT=off  OutDataTypeStr=boolean
  Product{,1..3} (4 alike) : Product
  SinCos : Trigonometry  Operator=sincos
  collided : Outport
  wires:
  Demux2/1 -> Add1/1
  OR/1 -> NOT/1
  c2/1 -> Demux2/1
  Add1/1 -> Product2/1, Product/1  "dx"
  SinCos/1 -> Product2/2, Product1/2  "s"
  Demux1/1 -> Add1/2  "point0"
  Abs1/1 -> Compare To Constant1/1
  Compare To Constant1/1 -> OR/2
  Demux1/2 -> Add/2  "point1"
  NOT/1 -> collided/1
  Abs/1 -> Compare To Constant/1
  Demux2/2 -> Add/1
  Product/1 -> Add2/1
  v1cor4/1 -> Demux1/1
  psi2/1 -> Gain/1
  Gain/1 -> SinCos/1
  Product2/1 -> Add3/1
  Product3/1 -> Add3/2
  Compare To Constant/1 -> OR/1
  SinCos/2 -> Product3/2, Product/2  "c"
  Add2/1 -> Abs/1  "rot_dx"
  Add3/1 -> Abs1/1  "rot_dy"
  Product1/1 -> Add2/2
  Add/1 -> Product1/1, Product3/1  "dy"

== system rlOvertakeTwoCars/Collision Detector/Subsystem8 ==
  psi1 : Inport
  c1 : Inport  Port=2
  v2cor1 : Inport  Port=3
  Abs : Abs  SaturateOnIntegerOverflow=off
  Abs1 : Abs  SaturateOnIntegerOverflow=off
  Add : Sum  Inputs=-+
  Add1 : Sum  Inputs=-+
  Add2 : Sum  Inputs=+-
  Add3 : Sum
  Compare To Constant : simulink/Logic and Bit Operations/Compare To Constant  relop=>  const=L/2  OutDataTypeStr=boolean
  Compare To Constant1 : simulink/Logic and Bit Operations/Compare To Constant  relop=>  const=W/2  OutDataTypeStr=boolean
  Demux1 : Demux  Outputs=2
  Demux2 : Demux  Outputs=2
  Gain : Gain  Gain=-1
  NOT : Logic  Operator=NOT  IconShape=distinctive  AllPortsSameDT=off  OutDataTypeStr=boolean
  OR : Logic  Operator=OR  IconShape=distinctive  AllPortsSameDT=off  OutDataTypeStr=boolean
  Product{,1..3} (4 alike) : Product
  SinCos : Trigonometry  Operator=sincos
  collided : Outport
  wires:
  Demux2/1 -> Add1/1
  OR/1 -> NOT/1
  c1/1 -> Demux2/1
  Add1/1 -> Product2/1, Product/1  "dx"
  SinCos/1 -> Product2/2, Product1/2  "s"
  Demux1/1 -> Add1/2  "point0"
  Abs1/1 -> Compare To Constant1/1
  Compare To Constant1/1 -> OR/2
  Demux1/2 -> Add/2  "point1"
  NOT/1 -> collided/1
  Abs/1 -> Compare To Constant/1
  Demux2/2 -> Add/1
  Product/1 -> Add2/1
  v2cor1/1 -> Demux1/1
  psi1/1 -> Gain/1
  Gain/1 -> SinCos/1
  Product2/1 -> Add3/1
  Product3/1 -> Add3/2
  Compare To Constant/1 -> OR/1
  SinCos/2 -> Product3/2, Product/2  "c"
  Add2/1 -> Abs/1  "rot_dx"
  Add3/1 -> Abs1/1  "rot_dy"
  Product1/1 -> Add2/2
  Add/1 -> Product1/1, Product3/1  "dy"

== system rlOvertakeTwoCars/Collision Detector/Subsystem9 ==
  psi1 : Inport
  c1 : Inport  Port=2
  v2cor2 : Inport  Port=3
  Abs : Abs  SaturateOnIntegerOverflow=off
  Abs1 : Abs  SaturateOnIntegerOverflow=off
  Add : Sum  Inputs=-+
  Add1 : Sum  Inputs=-+
  Add2 : Sum  Inputs=+-
  Add3 : Sum
  Compare To Constant : simulink/Logic and Bit Operations/Compare To Constant  relop=>  const=L/2  OutDataTypeStr=boolean
  Compare To Constant1 : simulink/Logic and Bit Operations/Compare To Constant  relop=>  const=W/2  OutDataTypeStr=boolean
  Demux1 : Demux  Outputs=2
  Demux2 : Demux  Outputs=2
  Gain : Gain  Gain=-1
  NOT : Logic  Operator=NOT  IconShape=distinctive  AllPortsSameDT=off  OutDataTypeStr=boolean
  OR : Logic  Operator=OR  IconShape=distinctive  AllPortsSameDT=off  OutDataTypeStr=boolean
  Product{,1..3} (4 alike) : Product
  SinCos : Trigonometry  Operator=sincos
  collided : Outport
  wires:
  Demux2/1 -> Add1/1
  OR/1 -> NOT/1
  c1/1 -> Demux2/1
  Add1/1 -> Product2/1, Product/1  "dx"
  SinCos/1 -> Product2/2, Product1/2  "s"
  Demux1/1 -> Add1/2  "point0"
  Abs1/1 -> Compare To Constant1/1
  Compare To Constant1/1 -> OR/2
  Demux1/2 -> Add/2  "point1"
  NOT/1 -> collided/1
  Abs/1 -> Compare To Constant/1
  Demux2/2 -> Add/1
  Product/1 -> Add2/1
  v2cor2/1 -> Demux1/1
  psi1/1 -> Gain/1
  Gain/1 -> SinCos/1
  Product2/1 -> Add3/1
  Product3/1 -> Add3/2
  Compare To Constant/1 -> OR/1
  SinCos/2 -> Product3/2, Product/2  "c"
  Add2/1 -> Abs/1  "rot_dx"
  Add3/1 -> Abs1/1  "rot_dy"
  Product1/1 -> Add2/2
  Add/1 -> Product1/1, Product3/1  "dy"

== system rlOvertakeTwoCars/MPC Based Controller/Pedal map ==
  note: This 2-D Lookup Table was created using a for-loop and then normalizing. This is required because the output of the MPC controller is acceleration (m/s^2), but the powertrain model uses pedal commands from 0-1.
      |
      | Here are the steps in the script to create the table:
      |
      | 1.) The for-loop is used to calculate the required torque (Nm) from the powertrain.
      | 2.) The positive torque values are normalized based on peak positive motor torque, and the negative torques are normalized based on the peak brake pressure. This results in a pedal map with values of -1 to 1.
      |
      | This map required two values to be calibrated.
      |
      | This is a simple linearized map, but this can be altered for better drivability.
  note: The saturation blocks ensure the acceleration limits are kept at ±1.
  note: The 'Dead Zone' blocks is used to ensure that the pedal command is zero.
  vx : Inport
  a : Inport  Port=2
  Dead Zone1 : DeadZone  LowerValue=-0.001  UpperValue=0.001
  Dead Zone2 : DeadZone  LowerValue=-0.001  UpperValue=0.001
  Gain : Gain  Gain=-1
  Pedal map : Lookup_n-D  BreakpointsForDimension1=vel_vec  BreakpointsForDimension2=accel_vec  Table=pedal_map'  InternalRulePriority=Speed  RndMeth=Simplest
      settings: InputPortMap=u0,u1
  Saturation : Saturate  UpperLimit=1  LowerLimit=0
  Saturation1 : Saturate  UpperLimit=0  LowerLimit=-1
  Out1 : Outport
  Out2 : Outport  Port=2
  wires:
  Pedal map/1 -> Saturation/1, Saturation1/1
  Saturation/1 -> Dead Zone1/1
  Saturation1/1 -> Gain/1
  Gain/1 -> Dead Zone2/1
  vx/1 -> Pedal map/1
  Dead Zone1/1 -> Out1/1
  Dead Zone2/1 -> Out2/1
  a/1 -> Pedal map/2

== system rlOvertakeTwoCars/MPC Based Controller/Sensor Dynamics ==
  Current curvature : Inport
  Longitudinal velocity : Inport  Port=2
  Lateral velocity : Inport  Port=3
  Yaw rate : Inport  Port=4
  Integrator : Integrator
  Integrator2 : Integrator
  Mux1 : Mux  Inputs=[1 1 1]
  Product : Product
  Subtract : Sum  Inputs=-+
  e1dot : Fcn  Expr=u(1)*u(3)+u(2)
  Lateral deviation : Outport  VectorParamsAs1DForOutWhenUnconnected=off
  Relative yaw angle : Outport  Port=2  VectorParamsAs1DForOutWhenUnconnected=off
  wires:
  Subtract/1 -> Integrator2/1  "e2dot"
  Yaw rate/1 -> Subtract/2
  Product/1 -> Subtract/1
  Integrator/1 -> Lateral deviation/1  "e1"
  Lateral velocity/1 -> Mux1/2
  Longitudinal velocity/1 -> Mux1/1, Product/1
  e1dot/1 -> Integrator/1
  Mux1/1 -> e1dot/1
  Integrator2/1 -> Relative yaw angle/1, Mux1/3  "e2"
  Current curvature/1 -> Product/2

== system rlOvertakeTwoCars/Obs // Reward 9-6/Overtaking ==
  note: Overtake on right sigmoid
  note: Overtaking reward sigmoid
  ry : Inport
  xgap : Inport  Port=2
  ygap : Inport  Port=3
  -k_D : Gain  Gain=-0.3
  -k_G : Gain  Gain=-1.2
  Add : Sum
  Add1 : Sum  Inputs=+-
  Add2 : Sum
  C : Gain  Gain=0
  Constant{,2..4} (4 alike) : Constant
  Constant1 : Constant  Value=0
  D : Gain  Gain=3
  Divide : Product  Inputs=*/
  Divide1 : Product  Inputs=*/
  Exp : Math
  Exp1 : Math
  G : Gain  Gain=0.25
  G1 : Constant  Value=0.25
  Slipstream reward enable : Switch  Criteria=u2 > Threshold  Threshold=-6.5  SaturateOnIntegerOverflow=off  InputSameDT=off
  Sum1 : Sum  Inputs=+++
  h : Constant  Value=-1
  switch2 : Switch  Criteria=u2 > Threshold  SaturateOnIntegerOverflow=off  InputSameDT=off
  r_ot : Outport  VectorParamsAs1DForOutWhenUnconnected=off
  wires:
  Constant1/1 -> Slipstream reward enable/1
  C/1 -> Slipstream reward enable/3
  Divide/1 -> D/1
  ry/1 -> C/1
  Slipstream reward enable/1 -> Sum1/1
  Sum1/1 -> r_ot/1
  D/1 -> Sum1/2
  Exp/1 -> Add/1
  Constant/1 -> Divide/1
  -k_D/1 -> Exp/1
  Constant2/1 -> Add/2
  Add/1 -> Divide/2
  Add1/1 -> -k_D/1
  h/1 -> Add1/2
  Constant4/1 -> Add2/2
  Add2/1 -> Divide1/2
  -k_G/1 -> Exp1/1
  Exp1/1 -> Add2/1
  Constant3/1 -> Divide1/1
  Divide1/1 -> G/1
  ygap/1 -> -k_G/1
  xgap/1 -> Slipstream reward enable/2, switch2/2, Add1/1
  G1/1 -> switch2/1
  G/1 -> switch2/3
  switch2/1 -> Sum1/3
